simulink model "k1vismce"  (Simulink 8.8)
settings: Solver=ode45  StartTime=0.0  StopTime=10.0  RelTol=1e-3  EnableMultiTasking=on
libraries: cdsIPCx x20, cdsEpicsOut x4, dac x2, cdsBit2Word x2, cdsFilt x2, cdsAdcx0 x1, cdsAdcx1 x1, cdsCDI64 x1, cdsCDO64 x1, PAYLOAD_MASTER x1, cdsEpicsBinIn x1, cdsWord2Bit x1
settings Model: SuppressorTable=22 serialization::archive 11 0 3 0 0 0 11 0  Creator=keiko  LastModifiedBy=controls
settings DataIOCC: SignalLoggingSaveFormat=Dataset
settings DebuggingCC: UnderspecifiedInitializationDetection=Simplified  MergeDetectMultiDrivingBlocksExec=error  SolverPrmCheckMsg=warning  FcnCallInpInsideContextMsg=error  AllowSymbolicDim=off  StateNameClashWarn=none
settings GRTTargetCC: CombineOutputUpdateFcns=on  GRTInterface=off

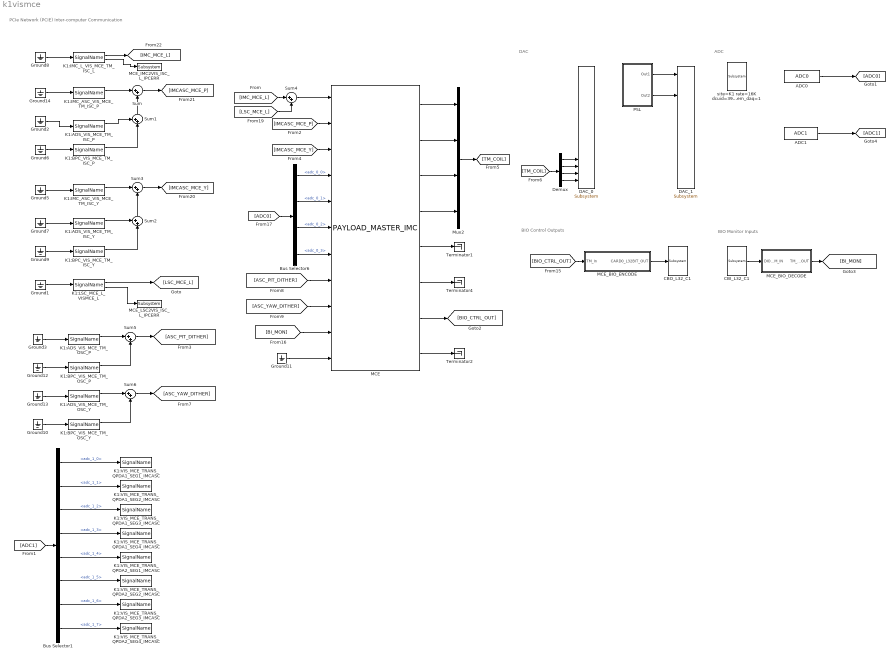
== system k1vismce ==
  note: PCIe Network (PCIE)
      | Inter-computer Communication
  note: DAC
  note: ADC
  note: BIO Control Outputs
  note: BIO Monitor Inputs
  ADC0 : cdsAdcx0/ADC0  Tag=cdsAdc  Description=|
      | type-GSC_16AI64SSA
      | card_num=0
      settings: AttributesFormatString=%<Description>\n%<Tag>
  ADC1 : cdsAdcx1/ADC1  Tag=cdsAdc  Description=|
      | type-GSC_16AI64SSA
      | card_num=1
      settings: AttributesFormatString=%<Description>\n%<Tag>
  Bus Selector1 : BusSelector  Description=ADC Selector  OutputSignals=adc_1_0,adc_1_1,adc_1_2,adc_1_3,adc_1_4,adc_1_5,adc_1_6,adc_1_7
      settings: AttributesFormatString=%<Description>
  Bus Selector6 : BusSelector  Description=ADC Selector  OutputSignals=adc_0_0,adc_0_1,adc_0_2,adc_0_3
      settings: AttributesFormatString=%<Description>
  CBI_L32_C1 : cdsCDI64/Subsystem  Tag=cdsCDI64  Description=card_num=2
      settings: AttributesFormatString=%<Tag>\n%<Description>
  CBO_L32_C1 : cdsCDO64/Subsystem  Tag=cdsCDO64  Description=card_num=2
      settings: AttributesFormatString=%<Tag>\n%<Description>
  DAC_0 : dac/Subsystem  Description=|
      | type=GSC_16AO16,
      | card_num=0
      settings: AttributesFormatString=%<Description>
  DAC_1 : dac/Subsystem  Description=|
      | type=GSC_16AO16,
      | card_num=1
      settings: AttributesFormatString=%<Description>
  Demux : Demux
  Ground{1..3,5..14} (13 alike) : Ground
  K1:ADS_VIS_MCE_TM_ISC_P : cdsIPCx/SignalName  Tag=cdsIPCx_PCIE  Description=Inter-Process Communication via PCI Express network.
      settings: AttributesFormatString=%<Tag>
  K1:ADS_VIS_MCE_TM_ISC_Y : cdsIPCx/SignalName  Tag=cdsIPCx_PCIE  Description=Inter-Process Communication via PCI Express network.
      settings: AttributesFormatString=%<Tag>
  K1:ADS_VIS_MCE_TM_OSC_P : cdsIPCx/SignalName  Tag=cdsIPCx_PCIE  Description=Inter-Process Communication via PCI Express network.
      settings: AttributesFormatString=%<Tag>
  K1:ADS_VIS_MCE_TM_OSC_Y : cdsIPCx/SignalName  Tag=cdsIPCx_PCIE  Description=Inter-Process Communication via PCI Express network.
      settings: AttributesFormatString=%<Tag>
  K1:BPC_VIS_MCE_TM_ISC_P : cdsIPCx/SignalName  Tag=cdsIPCx_PCIE  Description=Inter-Process Communication via PCI Express network.
      settings: AttributesFormatString=%<Tag>
  K1:BPC_VIS_MCE_TM_ISC_Y : cdsIPCx/SignalName  Tag=cdsIPCx_PCIE  Description=Inter-Process Communication via PCI Express network.
      settings: AttributesFormatString=%<Tag>
  K1:BPC_VIS_MCE_TM_OSC_P : cdsIPCx/SignalName  Tag=cdsIPCx_PCIE  Description=Inter-Process Communication via PCI Express network.
      settings: AttributesFormatString=%<Tag>
  K1:BPC_VIS_MCE_TM_OSC_Y : cdsIPCx/SignalName  Tag=cdsIPCx_PCIE  Description=Inter-Process Communication via PCI Express network.
      settings: AttributesFormatString=%<Tag>
  K1:IMC_ASC_VIS_MCE_TM_ISC_P : cdsIPCx/SignalName  Tag=cdsIPCx_PCIE  Description=Inter-Process Communication via PCI Express network.
      settings: AttributesFormatString=%<Tag>
  K1:IMC_ASC_VIS_MCE_TM_ISC_Y : cdsIPCx/SignalName  Tag=cdsIPCx_PCIE  Description=Inter-Process Communication via PCI Express network.
      settings: AttributesFormatString=%<Tag>
  K1:IMC_L_VIS_MCE_TM_ISC_L : cdsIPCx/SignalName  Tag=cdsIPCx_PCIE  Description=Inter-Process Communication via PCI Express network.
      settings: AttributesFormatString=%<Tag>
  K1:LSC_MCE_L_VISMCE_L : cdsIPCx/SignalName  Tag=cdsIPCx_PCIE  Description=Inter-Process Communication via PCI Express network.
      settings: AttributesFormatString=%<Tag>
  K1:VIS_MCE_TRANS_QPDA1_SEG1_IMCASC : cdsIPCx/SignalName  Tag=cdsIPCx_PCIE  Description=Inter-Process Communication via PCI Express network.
      settings: AttributesFormatString=%<Tag>
  K1:VIS_MCE_TRANS_QPDA1_SEG2_IMCASC : cdsIPCx/SignalName  Tag=cdsIPCx_PCIE  Description=Inter-Process Communication via PCI Express network.
      settings: AttributesFormatString=%<Tag>
  K1:VIS_MCE_TRANS_QPDA1_SEG3_IMCASC : cdsIPCx/SignalName  Tag=cdsIPCx_PCIE  Description=Inter-Process Communication via PCI Express network.
      settings: AttributesFormatString=%<Tag>
  K1:VIS_MCE_TRANS_QPDA1_SEG4_IMCASC : cdsIPCx/SignalName  Tag=cdsIPCx_PCIE  Description=Inter-Process Communication via PCI Express network.
      settings: AttributesFormatString=%<Tag>
  K1:VIS_MCE_TRANS_QPDA2_SEG1_IMCASC : cdsIPCx/SignalName  Tag=cdsIPCx_PCIE  Description=Inter-Process Communication via PCI Express network.
      settings: AttributesFormatString=%<Tag>
  K1:VIS_MCE_TRANS_QPDA2_SEG2_IMCASC : cdsIPCx/SignalName  Tag=cdsIPCx_PCIE  Description=Inter-Process Communication via PCI Express network.
      settings: AttributesFormatString=%<Tag>
  K1:VIS_MCE_TRANS_QPDA2_SEG3_IMCASC : cdsIPCx/SignalName  Tag=cdsIPCx_PCIE  Description=Inter-Process Communication via PCI Express network.
      settings: AttributesFormatString=%<Tag>
  K1:VIS_MCE_TRANS_QPDA2_SEG4_IMCASC : cdsIPCx/SignalName  Tag=cdsIPCx_PCIE  Description=Inter-Process Communication via PCI Express network.
      settings: AttributesFormatString=%<Tag>
  MCE : PAYLOAD_MASTER/PAYLOAD_MASTER_IMC  Description=TYPEC SINGLE MASTER
      settings: AttributesFormatString=%<Description>
  MCE_BIO_DECODE : Subsystem
  MCE_BIO_ENCODE : Subsystem
  MCE_IMC2VIS_ISC_L_IPCERR : cdsEpicsOut/Subsystem  Tag=cdsEpicsOutput  Description=|
      | Purpose:                                          
      | Output a FE signal to an EPICS channel.           
      |                                                   
      | Operation:                                        
      | Takes input value and passes it to EPICS record.  
      |                                                   
      | Usage:                                            
      | Name the part with the desired EPICS rrecord name.
      settings: AttributesFormatString=%<Tag>
  MCE_LSC2VIS_ISC_L_IPCERR : cdsEpicsOut/Subsystem  Tag=cdsEpicsOutput  Description=|
      | Purpose:                                          
      | Output a FE signal to an EPICS channel.           
      |                                                   
      | Operation:                                        
      | Takes input value and passes it to EPICS record.  
      |                                                   
      | Usage:                                            
      | Name the part with the desired EPICS rrecord name.
      settings: AttributesFormatString=%<Tag>
  Mux2 : Mux
  PSL : Subsystem  Tag=top_names
  Sum{,3..6} (5 alike) : Sum  Inputs=|++
  Sum1 : Sum  Inputs=++|
  Sum2 : Sum  Inputs=++|
  Terminator1 : Terminator
  Terminator2 : Terminator
  Terminator4 : Terminator
  site=K1 rate=16K dcuid=39 host=k1imc0 specific_cpu=3 adcSlave=1 shmem_daq=1 : cdsParameters/Subsystem  Tag=cdsParameters  Description=|
      | Purpose:                                                                                                                                                                                                                                
      | Provide system parameters to the FE code generator to properly configure the generated EPICS names, rep rate of the FE controller, and the Data Acquisition node ID for proper storage of data from this FE controller.                 
      |                                                                                                                                                                                                                                         
      | Useage:                                                                                                                                                                                                                                 
      | The part NAME field is used to identify the FE parameters. It must be of the form:                                                                                                                                                      
      | site=                                                                                                                                                                                                                                   
      | rate=                                                                                                                                                                                                                                   
      | dcuid=                                                                                                                                                                                                                                  
      |                                                                                                                                                                                                                                         
      | Where:                                                                                                                                                                                                                                  
      | site= argument may be H1, H2, L1, M1, G1, either as a single argument or multiple, for example site=H1,H2. These are the only names allowed. These will become the first two characters of all EPICS and signal names (for example G1:).
      |                                                                                                                                                                                                                                         
      | rate= may be 2K, 16K, 32K, or 64K                                                                                                                                                                                                       
      |                                                                                                                                                                                                                                         
      | dcuid= is site specific ie it must be unique at each site.
      settings: AttributesFormatString=%<Tag>
  wires:
  ADC0/1 -> [ADC0]
  [BI_MON] -> MCE/10
  Ground11/1 -> MCE/11
  MCE/2 -> Mux2/2
  MCE/3 -> Mux2/3
  Mux2/1 -> [TM_COIL]
  MCE/1 -> Mux2/1
  MCE/4 -> Mux2/4
  [TM_COIL] -> Demux/1
  Demux/1 -> DAC_0/13
  Demux/2 -> DAC_0/14
  Demux/3 -> DAC_0/15
  Demux/4 -> DAC_0/16
  Bus Selector6/1 -> MCE/4  "<adc_0_0>"
  Bus Selector6/2 -> MCE/5  "<adc_0_1>"
  Bus Selector6/3 -> MCE/6  "<adc_0_2>"
  Bus Selector6/4 -> MCE/7  "<adc_0_3>"
  [IMCASC_MCE_Y] -> MCE/3
  [IMCASC_MCE_P] -> MCE/2
  MCE/5 -> Terminator1/1
  MCE/6 -> Terminator4/1
  Bus Selector1/2 -> K1:VIS_MCE_TRANS_QPDA1_SEG2_IMCASC/1  "<adc_1_1>"
  Bus Selector1/3 -> K1:VIS_MCE_TRANS_QPDA1_SEG3_IMCASC/1  "<adc_1_2>"
  Bus Selector1/4 -> K1:VIS_MCE_TRANS_QPDA1_SEG4_IMCASC/1  "<adc_1_3>"
  Bus Selector1/1 -> K1:VIS_MCE_TRANS_QPDA1_SEG1_IMCASC/1  "<adc_1_0>"
  ADC1/1 -> [ADC1]
  Bus Selector1/5 -> K1:VIS_MCE_TRANS_QPDA2_SEG1_IMCASC/1  "<adc_1_4>"
  Bus Selector1/6 -> K1:VIS_MCE_TRANS_QPDA2_SEG2_IMCASC/1  "<adc_1_5>"
  Bus Selector1/7 -> K1:VIS_MCE_TRANS_QPDA2_SEG3_IMCASC/1  "<adc_1_6>"
  Bus Selector1/8 -> K1:VIS_MCE_TRANS_QPDA2_SEG4_IMCASC/1  "<adc_1_7>"
  MCE_BIO_DECODE/1(TM_BIO_OUT) -> [BI_MON]
  CBI_L32_C1/1 -> MCE_BIO_DECODE/1(DIO_TM_IN)
  [BIO_CTRL_OUT] -> MCE_BIO_ENCODE/1(TM_In)
  MCE_BIO_ENCODE/1(CARD0_L32BIT_OUT) -> CBO_L32_C1/1
  MCE/7 -> [BIO_CTRL_OUT]
  [IMC_MCE_L] -> Sum4/1
  [LSC_MCE_L] -> Sum4/2
  Sum4/1 -> MCE/1
  PSL/2(Out2) -> DAC_1/4
  PSL/1(Out1) -> DAC_1/1
  K1:IMC_L_VIS_MCE_TM_ISC_L/2 -> MCE_IMC2VIS_ISC_L_IPCERR/1
  Ground8/1 -> K1:IMC_L_VIS_MCE_TM_ISC_L/1
  K1:IMC_L_VIS_MCE_TM_ISC_L/1 -> [IMC_MCE_L]
  Ground14/1 -> K1:IMC_ASC_VIS_MCE_TM_ISC_P/1
  Ground5/1 -> K1:IMC_ASC_VIS_MCE_TM_ISC_Y/1
  Ground2/1 -> K1:ADS_VIS_MCE_TM_ISC_P/1
  K1:IMC_ASC_VIS_MCE_TM_ISC_P/1 -> Sum/1
  Sum/1 -> [IMCASC_MCE_P]
  Sum1/1 -> Sum/2
  K1:ADS_VIS_MCE_TM_ISC_P/1 -> Sum1/1
  Ground6/1 -> K1:BPC_VIS_MCE_TM_ISC_P/1
  K1:BPC_VIS_MCE_TM_ISC_P/1 -> Sum1/2
  Ground7/1 -> K1:ADS_VIS_MCE_TM_ISC_Y/1
  K1:ADS_VIS_MCE_TM_ISC_Y/1 -> Sum2/1
  Ground9/1 -> K1:BPC_VIS_MCE_TM_ISC_Y/1
  K1:BPC_VIS_MCE_TM_ISC_Y/1 -> Sum2/2
  K1:IMC_ASC_VIS_MCE_TM_ISC_Y/1 -> Sum3/1
  Sum3/1 -> [IMCASC_MCE_Y]
  Sum2/1 -> Sum3/2
  K1:ADS_VIS_MCE_TM_OSC_P/1 -> Sum5/1
  K1:BPC_VIS_MCE_TM_OSC_P/1 -> Sum5/2
  Ground3/1 -> K1:ADS_VIS_MCE_TM_OSC_P/1
  Ground12/1 -> K1:BPC_VIS_MCE_TM_OSC_P/1
  Ground13/1 -> K1:ADS_VIS_MCE_TM_OSC_Y/1
  Ground10/1 -> K1:BPC_VIS_MCE_TM_OSC_Y/1
  K1:ADS_VIS_MCE_TM_OSC_Y/1 -> Sum6/1
  K1:BPC_VIS_MCE_TM_OSC_Y/1 -> Sum6/2
  Sum6/1 -> [ASC_YAW_DITHER]
  Ground1/1 -> K1:LSC_MCE_L_VISMCE_L/1
  K1:LSC_MCE_L_VISMCE_L/2 -> MCE_LSC2VIS_ISC_L_IPCERR/1
  K1:LSC_MCE_L_VISMCE_L/1 -> [LSC_MCE_L]
  [ADC0] -> Bus Selector6/1
  ? -> DAC_0/7
  MCE/8 -> Terminator2/1
  [ADC1] -> Bus Selector1/1
  Sum5/1 -> [ASC_PIT_DITHER]
  [ASC_PIT_DITHER] -> MCE/8
  [ASC_YAW_DITHER] -> MCE/9

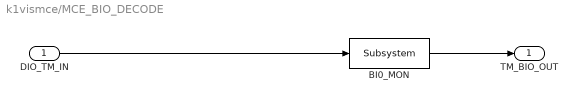
== system k1vismce/MCE_BIO_DECODE ==
  DIO_TM_IN : Inport
  BI0_MON : cdsEpicsOut/Subsystem  Tag=cdsEpicsOutput  Description=|
      | Purpose:                                          
      | Output a FE signal to an EPICS channel.           
      |                                                   
      | Operation:                                        
      | Takes input value and passes it to EPICS record.  
      |                                                   
      | Usage:                                            
      | Name the part with the desired EPICS rrecord name.
      settings: AttributesFormatString=%<Tag>
  TM_BIO_OUT : Outport
  wires:
  DIO_TM_IN/1 -> BI0_MON/1
  BI0_MON/1 -> TM_BIO_OUT/1

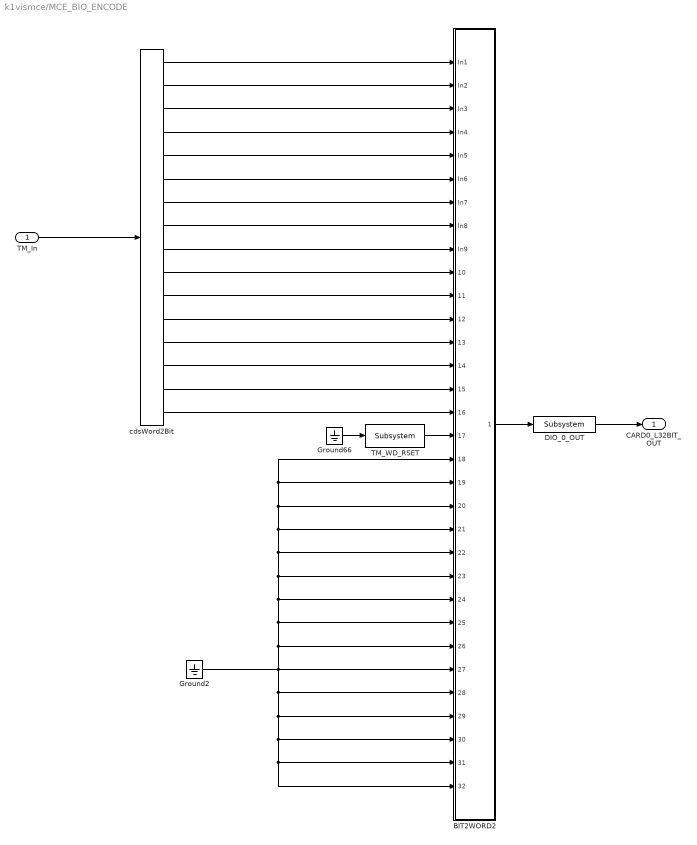
== system k1vismce/MCE_BIO_ENCODE ==
  TM_In : Inport
  BIT2WORD2 : Subsystem
  DIO_0_OUT : cdsEpicsOut/Subsystem  Tag=cdsEpicsOutput  Description=|
      | Purpose:                                          
      | Output a FE signal to an EPICS channel.           
      |                                                   
      | Operation:                                        
      | Takes input value and passes it to EPICS record.  
      |                                                   
      | Usage:                                            
      | Name the part with the desired EPICS rrecord name.
      settings: AttributesFormatString=%<Tag>
  Ground2 : Ground
  Ground66 : Ground
  TM_WD_RSET : cdsEpicsBinIn/Subsystem  Tag=cdsEpicsBinIn  Description=|
      | Purpose:                                                                            
      | Create an EPICS binary (0 or 1) input channel to the FE realtime controls.          
      |                                                                                     
      | Operation:                                                                          
      | Outputs value from an EPICS ai record. Value is binary input (bi Epics record type).
      |                                                                                     
      | Usage:                                                                              
      | Name the part with the desired EPICS channel name.
      settings: AttributesFormatString=%<Tag>
  cdsWord2Bit : cdsWord2Bit/cdsWord2Bit  Tag=cdsWord2Bit  Description=Generate 16 0/1 outputs from single 16-bit integer input
      settings: AttributesFormatString=cdsWord2Bit
  CARD0_L32BIT_OUT : Outport
  wires:
  Ground2/1 -> BIT2WORD2/20(In20), BIT2WORD2/18(In18), BIT2WORD2/19(In19), BIT2WORD2/21(In21), BIT2WORD2/22(In22), BIT2WORD2/23(In23), BIT2WORD2/24(In24), BIT2WORD2/25(In25), BIT2WORD2/26(In26), BIT2WORD2/28(In28), BIT2WORD2/31(In31), BIT2WORD2/32(In32), BIT2WORD2/30(In30), BIT2WORD2/29(In29), BIT2WORD2/27(In27)
  TM_In/1 -> cdsWord2Bit/1
  cdsWord2Bit/4 -> BIT2WORD2/4(In4)
  cdsWord2Bit/5 -> BIT2WORD2/5(In5)
  cdsWord2Bit/3 -> BIT2WORD2/3(In3)
  cdsWord2Bit/2 -> BIT2WORD2/2(In2)
  cdsWord2Bit/6 -> BIT2WORD2/6(In6)
  cdsWord2Bit/1 -> BIT2WORD2/1(In1)
  cdsWord2Bit/7 -> BIT2WORD2/7(In7)
  cdsWord2Bit/8 -> BIT2WORD2/8(In8)
  cdsWord2Bit/9 -> BIT2WORD2/9(In9)
  cdsWord2Bit/10 -> BIT2WORD2/10(In10)
  cdsWord2Bit/11 -> BIT2WORD2/11(In11)
  Ground66/1 -> TM_WD_RSET/1
  TM_WD_RSET/1 -> BIT2WORD2/17(In17)
  DIO_0_OUT/1 -> CARD0_L32BIT_OUT/1
  BIT2WORD2/1(Out1) -> DIO_0_OUT/1
  cdsWord2Bit/12 -> BIT2WORD2/12(In12)
  cdsWord2Bit/13 -> BIT2WORD2/13(In13)
  cdsWord2Bit/14 -> BIT2WORD2/14(In14)
  cdsWord2Bit/15 -> BIT2WORD2/15(In15)
  cdsWord2Bit/16 -> BIT2WORD2/16(In16)

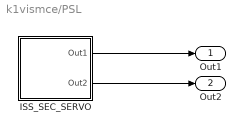
== system k1vismce/PSL ==
  ISS_SEC_SERVO : Subsystem
  Out1 : Outport
  Out2 : Outport  Port=2
  wires:
  ISS_SEC_SERVO/1(Out1) -> Out1/1
  ISS_SEC_SERVO/2(Out2) -> Out2/1

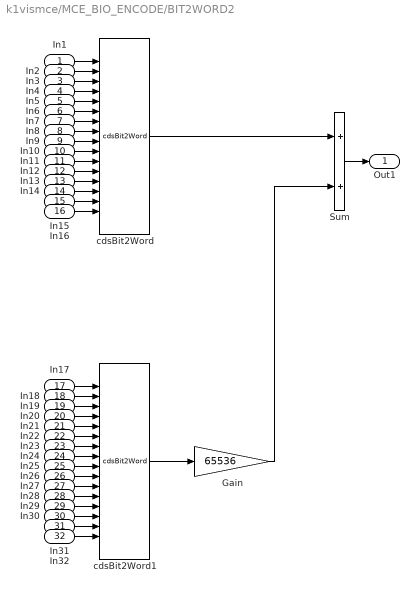
== system k1vismce/MCE_BIO_ENCODE/BIT2WORD2 ==
  In1 : Inport
  In2 : Inport  Port=2
  In3 : Inport  Port=3
  In4 : Inport  Port=4
  In5 : Inport  Port=5
  In6 : Inport  Port=6
  In7 : Inport  Port=7
  In8 : Inport  Port=8
  In9 : Inport  Port=9
  In10 : Inport  Port=10
  In11 : Inport  Port=11
  In12 : Inport  Port=12
  In13 : Inport  Port=13
  In14 : Inport  Port=14
  In15 : Inport  Port=15
  In16 : Inport  Port=16
  In17 : Inport  Port=17
  In18 : Inport  Port=18
  In19 : Inport  Port=19
  In20 : Inport  Port=20
  In21 : Inport  Port=21
  In22 : Inport  Port=22
  In23 : Inport  Port=23
  In24 : Inport  Port=24
  In25 : Inport  Port=25
  In26 : Inport  Port=26
  In27 : Inport  Port=27
  In28 : Inport  Port=28
  In29 : Inport  Port=29
  In30 : Inport  Port=30
  In31 : Inport  Port=31
  In32 : Inport  Port=32
  Gain : Gain  Gain=65536
  Sum : Sum
  cdsBit2Word : cdsBit2Word/cdsBit2Word  Tag=cdsBit2Word  Description=Forms single 16 bit integer from 16 0/1 inputs.
      settings: AttributesFormatString=%<Tag>
  cdsBit2Word1 : cdsBit2Word/cdsBit2Word  Tag=cdsBit2Word  Description=Forms single 16 bit integer from 16 0/1 inputs.
      settings: AttributesFormatString=%<Tag>
  Out1 : Outport
  wires:
  Gain/1 -> Sum/2
  cdsBit2Word1/1 -> Gain/1
  cdsBit2Word/1 -> Sum/1
  In1/1 -> cdsBit2Word/1
  In2/1 -> cdsBit2Word/2
  In3/1 -> cdsBit2Word/3
  In4/1 -> cdsBit2Word/4
  In5/1 -> cdsBit2Word/5
  In6/1 -> cdsBit2Word/6
  In7/1 -> cdsBit2Word/7
  In8/1 -> cdsBit2Word/8
  In9/1 -> cdsBit2Word/9
  In10/1 -> cdsBit2Word/10
  Sum/1 -> Out1/1
  In11/1 -> cdsBit2Word/11
  In12/1 -> cdsBit2Word/12
  In13/1 -> cdsBit2Word/13
  In14/1 -> cdsBit2Word/14
  In15/1 -> cdsBit2Word/15
  In16/1 -> cdsBit2Word/16
  In17/1 -> cdsBit2Word1/1
  In18/1 -> cdsBit2Word1/2
  In19/1 -> cdsBit2Word1/3
  In20/1 -> cdsBit2Word1/4
  In21/1 -> cdsBit2Word1/5
  In22/1 -> cdsBit2Word1/6
  In23/1 -> cdsBit2Word1/7
  In24/1 -> cdsBit2Word1/8
  In25/1 -> cdsBit2Word1/9
  In26/1 -> cdsBit2Word1/10
  In27/1 -> cdsBit2Word1/11
  In28/1 -> cdsBit2Word1/12
  In29/1 -> cdsBit2Word1/13
  In30/1 -> cdsBit2Word1/14
  In31/1 -> cdsBit2Word1/15
  In32/1 -> cdsBit2Word1/16

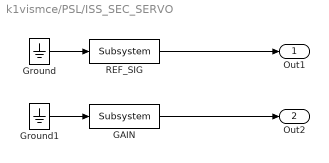
== system k1vismce/PSL/ISS_SEC_SERVO ==
  GAIN : cdsFilt/Subsystem  Tag=cdsFilt  Description=|
      | Purpose:                                                                                                                                                                                                                                  
      | Standard CDS IIR filter module.                                                                                                                                                                                                           
      |                                                                                                                                                                                                                                           
      | Operation:                                                                                                                                                                                                                                
      | Consists of 10 second order section IIR filters, plus a ramped gain stage. In FE code, also provides pre-defined test points and excitation channel inputs. The filter coefficients are defined in the LIGO system using the 'foton' tool.
      |                                                                                                                                                                                                                                           
      | Usage:                                                                                                                                                                                                                                    
      | Name the part with the desired filter module name.
      settings: AttributesFormatString=%<Tag>
  Ground : Ground
  Ground1 : Ground
  REF_SIG : cdsFilt/Subsystem  Tag=cdsFilt  Description=|
      | Purpose:                                                                                                                                                                                                                                  
      | Standard CDS IIR filter module.                                                                                                                                                                                                           
      |                                                                                                                                                                                                                                           
      | Operation:                                                                                                                                                                                                                                
      | Consists of 10 second order section IIR filters, plus a ramped gain stage. In FE code, also provides pre-defined test points and excitation channel inputs. The filter coefficients are defined in the LIGO system using the 'foton' tool.
      |                                                                                                                                                                                                                                           
      | Usage:                                                                                                                                                                                                                                    
      | Name the part with the desired filter module name.
      settings: AttributesFormatString=%<Tag>
  Out1 : Outport
  Out2 : Outport  Port=2
  wires:
  REF_SIG/1 -> Out1/1
  GAIN/1 -> Out2/1
  Ground/1 -> REF_SIG/1
  Ground1/1 -> GAIN/1
